simulink model "L4_SIM"  (R2018a)
settings: Solver=ode1  StartTime=0.0  StopTime=60  FixedStep=GLB_FIXED_STEP_SIZE_CPV  RelTol=1e-3  EnableMultiTasking=on
undefined symbols (not defined in the file or in its folder): Cf, Chassis, Cr, CYCLE_ACC1_2A__AdaptiveCruiseCtrlMode, CYCLE_ACC1_2A__AdaptiveCruiseCtrlSetSpeed, CYCLE_CCVS1_00__CruiseCtrlSetSpeed, CYCLE_CCVS1_00__WheelBasedVehicleSpeed, CYCLE_EEC1_00__EngSpeed, CYCLE_ETC1_00__TransDrivelineEngaged, CYCLE_ETC2_00__TransActualGearRatio, CYCLE_ETC7_03__TransMode1Indicator, CYCLE_GPS_Latitude, CYCLE_GPS_Longitude, CYCLE_LFE1_00__EngFuelRate, CYCLE_Net_Engine_Percent_Torque, CYCLE_SSI2_03__PitchAngleExRange, CYCLE_TIME, CYCLE_UTM_Origin_X, CYCLE_UTM_Origin_Y, CYCLE_Vehicle_Distance, DiscIntNeverNeededParam, ENUM_J1939_PCC_STATE_T, ENUM_J1939_SWITCH_T, ENUM_STEERING_WHEEL_ANGLE_SENSOR_TYPE_T, GLB_FIXED_STEP_SIZE_CPV, GLB_TRANS_LOSS_TRQ_GEAR_STEP_MPV, GLB_TRANS_LOSS_TRQ_SPD_STEP_MPV, GLB_TRANS_LOSS_TRQ_TABLE_DATA_MPV, GLB_TRANS_LOSS_TRQ_TRQ_STEP_MPV, GLB_VEHICLE_CONFIG_ACCEL_PED_GATEWAY_APV, heading_0, Iz, L4_Controller, lf, lr, position_0, ptc_matlab_lib, STEERCTRL_10ms, SUB_ECU_L4_MABX, SUB_L4_Task_10ms, SUB_L4_Task_10ms_SUB_STEERCTRL, SUB_PLANT_Chassis, Task_10ms, Vx_0
libraries: EmE_MBD_Blockset x81, PTC_MBDS_LIB x71, simulink x38, simulink_extras x1, SUB_L4_Task_10000ms x1, SUB_L4_Task_1000ms x1, SUB_L4_Task_100ms x1, SUB_L4_Task_10ms_SUB_APTC x1, SUB_L4_Task_10ms_SUB_BRKPEDARB x1, SUB_L4_Task_10ms_SUB_FAULT_MANAGER x1, SUB_L4_Task_10ms_SUB_STATE_CONTROL x1, simulink_need_slupdate x1
(part 5 of 6)

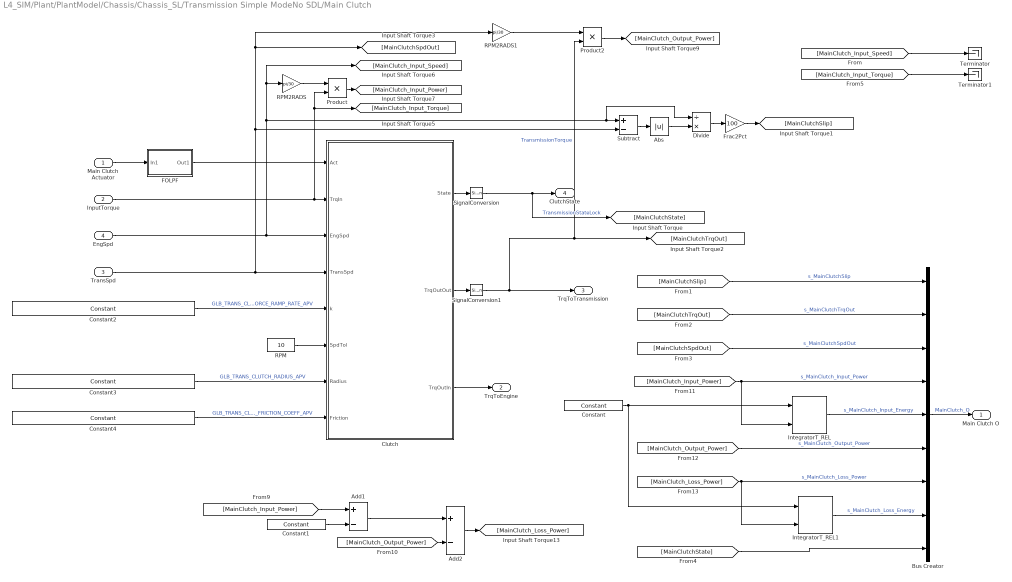
== system L4_SIM/Plant/PlantModel/Chassis/Chassis_SL/Transmission Simple ModeNo SDL/Main Clutch ==
  Main Clutch Actuator : Inport
  InputTorque : Inport  Port=2
  TransSpd : Inport  Port=3
  EngSpd : Inport  Port=4
  Abs : Abs
  Add1 : Sum  Inputs=+-
  Add2 : Sum  Inputs=+-
  Bus Creator : BusCreator  Inputs=9
  Clutch : Stateflow chart  TreatAsAtomicUnit=on
  Constant : PTC_MBDS_LIB/Extras/Sources/Constant  Value2=1  PTC_MBDS_BlockVersion=5.41  PTC_BlockType=PTC_MBDS_Constant
      settings: SourceProductName=PACCAR Technical Center MBDS Library
  Constant1 : PTC_MBDS_LIB/Extras/Sources/Constant  Value2=0  PTC_MBDS_BlockVersion=5.41  PTC_BlockType=PTC_MBDS_Constant
      settings: SourceProductName=PACCAR Technical Center MBDS Library
  Constant2 : PTC_MBDS_LIB/Extras/Sources/Constant  Value2=GLB_TRANS_CLUTCH_FORCE_RAMP_RATE_APV  PTC_MBDS_BlockVersion=5.41  PTC_BlockType=PTC_MBDS_Constant
      settings: SourceProductName=PACCAR Technical Center MBDS Library
      settings: AttributesFormatString=|
      | Value: 5000
      | Unit: 'N/s'
  Constant3 : PTC_MBDS_LIB/Extras/Sources/Constant  Value2=GLB_TRANS_CLUTCH_RADIUS_APV  PTC_MBDS_BlockVersion=5.41  PTC_BlockType=PTC_MBDS_Constant
      settings: SourceProductName=PACCAR Technical Center MBDS Library
      settings: AttributesFormatString=|
      | Value: 0.215
      | Unit: 'm'
  Constant4 : PTC_MBDS_LIB/Extras/Sources/Constant  Value2=GLB_TRANS_CLUTCH_FRICTION_COEFF_APV  PTC_MBDS_BlockVersion=5.41  PTC_BlockType=PTC_MBDS_Constant
      settings: SourceProductName=PACCAR Technical Center MBDS Library
      settings: AttributesFormatString=|
      | Value: 0.3
      | Unit: '1'
  Divide : Product  Inputs=/*
  FOLPF : Subsystem
  Frac2Pct : Gain  Gain=100
  IntegratorT_REL : PTC_MBDS_LIB/MBDS Standard Library/Extended Operations/Integrators/IntegratorT_REL  MXMN_Enabled=off  MX=Inf  MN=-Inf  dT_Enabled=off  dT=GLB_FIXED_STEP_SIZE_CPV  E_Enabled=off  R_Enabled=off  IV_Enabled=off  IV=0  B_min_Enabled=off  B_max_Enabled=off  PTC_MBDS_BlockVersion=5.41  PTC_BlockType=PTC_MBDS_IntegratorT_REL
      settings: SourceProductName=PACCAR Technical Center MBDS Library
      settings: AttributesFormatString=|
      | IV = %<IV>
      | MN = %<MN>
      | MX = %<MX>
      | dT = %<dT>
  IntegratorT_REL1 : PTC_MBDS_LIB/MBDS Standard Library/Extended Operations/Integrators/IntegratorT_REL  MXMN_Enabled=off  MX=Inf  MN=-Inf  dT_Enabled=off  dT=GLB_FIXED_STEP_SIZE_CPV  E_Enabled=off  R_Enabled=off  IV_Enabled=off  IV=0  B_min_Enabled=off  B_max_Enabled=off  PTC_MBDS_BlockVersion=5.41  PTC_BlockType=PTC_MBDS_IntegratorT_REL
      settings: SourceProductName=PACCAR Technical Center MBDS Library
      settings: AttributesFormatString=|
      | IV = %<IV>
      | MN = %<MN>
      | MX = %<MX>
      | dT = %<dT>
  Product : Product  RndMeth=Zero
  Product2 : Product  RndMeth=Zero
  RPM : Constant  Value=10
  RPM2RADS : Gain  Gain=pi/30
  RPM2RADS1 : Gain  Gain=pi/30
  SignalConversion : SignalConversion  ConversionOutput=Contiguous copy  OverrideOpt=off
  SignalConversion1 : SignalConversion  ConversionOutput=Contiguous copy  OverrideOpt=off
  Subtract : Sum  Inputs=+-
  Terminator : Terminator
      settings: InitFcn=|
      | try
      |    MBDS_BlockCallback('Update', gcb);
      | end
  Terminator1 : Terminator
      settings: InitFcn=|
      | try
      |    MBDS_BlockCallback('Update', gcb);
      | end
  Main Clutch O : Outport
  TrqToEngine : Outport  Port=2
  TrqToTransmission : Outport  Port=3
  ClutchState : Outport  Port=4
  wires:
  Constant2/1 -> Clutch/5(k)  "GLB_TRANS_CLUTCH_FORCE_RAMP_RATE_APV"
  SignalConversion1/1 -> TrqToTransmission/1, [MainClutchTrqOut], Product2/2  "TransmissionTorque"
  SignalConversion/1 -> [MainClutchState], ClutchState/1  "TransmissionStateLock"
  [MainClutch_Input_Torque] -> Terminator1/1
  [MainClutch_Input_Speed] -> Terminator/1
  [MainClutchState] -> Bus Creator/9
  Constant1/1 -> Add1/2
  Constant/1 -> IntegratorT_REL/1, IntegratorT_REL1/1
  Constant3/1 -> Clutch/7(Radius)  "GLB_TRANS_CLUTCH_RADIUS_APV"
  Constant4/1 -> Clutch/8(Friction)  "GLB_TRANS_CLUTCH_FRICTION_COEFF_APV"
  TransSpd/1 -> [MainClutchSpdOut], RPM2RADS1/1, Subtract/2, Clutch/4(TransSpd)
  Subtract/1 -> Abs/1
  Abs/1 -> Divide/2
  Divide/1 -> Frac2Pct/1
  RPM2RADS1/1 -> Product2/1
  RPM2RADS/1 -> Product/1
  Clutch/1(State) -> SignalConversion/1
  FOLPF/1(Out1) -> Clutch/1(Act)
  RPM/1 -> Clutch/6(SpdTol)
  EngSpd/1 -> RPM2RADS/1, [MainClutch_Input_Speed], Subtract/1, Divide/1, Clutch/3(EngSpd)
  InputTorque/1 -> [MainClutch_Input_Torque], Product/2, Clutch/2(TrqIn)
  Clutch/2(TrqOutOut) -> SignalConversion1/1
  Clutch/3(TrqOutIn) -> TrqToEngine/1
  Frac2Pct/1 -> [MainClutchSlip]
  [MainClutchSpdOut] -> Bus Creator/3  "s_MainClutchSpdOut"
  [MainClutchTrqOut] -> Bus Creator/2  "s_MainClutchTrqOut"
  [MainClutchSlip] -> Bus Creator/1  "s_MainClutchSlip"
  Bus Creator/1 -> Main Clutch O/1  "MainClutch_O"
  Main Clutch Actuator/1 -> FOLPF/1(In1)
  Product/1 -> [MainClutch_Input_Power]
  Product2/1 -> [MainClutch_Output_Power]
  [MainClutch_Input_Power] -> Add1/1
  [MainClutch_Output_Power] -> Add2/2
  Add1/1 -> Add2/1
  Add2/1 -> [MainClutch_Loss_Power]
  [MainClutch_Input_Power] -> Bus Creator/4, IntegratorT_REL/2  "s_MainClutch_Input_Power"
  [MainClutch_Output_Power] -> Bus Creator/6  "s_MainClutch_Output_Power"
  [MainClutch_Loss_Power] -> Bus Creator/7, IntegratorT_REL1/2  "s_MainClutch_Loss_Power"
  IntegratorT_REL1/1 -> Bus Creator/8  "s_MainClutch_Loss_Energy"
  IntegratorT_REL/1 -> Bus Creator/5  "s_MainClutch_Input_Energy"

== system L4_SIM/Controllers/Operator/Subsystem/SpdControlBrake/SpdControlBrake/PID/AntiWindup ==
  note: NOTE: THE ANTI-WINDUP FOR BRAKE IS THE SAME AS FOR TRACTION EXCEPT
      | FOR THE SAT_STATE LOGIC
  I_update : Inport
  Sat_state : Inport  Port=2
  Constant : Constant  Value=0
  Constant1 : Constant  Value=-1
  Constant2 : Constant
  Constant3 : Constant
  Constant4 : Constant  Value=-1
  Constant5 : Constant  Value=2
  Logical Operator : Logic  Operator=OR  AllPortsSameDT=off  OutDataTypeStr=boolean
  Logical Operator1 : Logic  AllPortsSameDT=off  OutDataTypeStr=boolean
  Logical Operator2 : Logic  AllPortsSameDT=off  OutDataTypeStr=boolean
  Logical Operator3 : Logic  AllPortsSameDT=off  OutDataTypeStr=boolean
  Relational Operator1 : RelationalOperator  Operator=~=  OutDataTypeStr=boolean  RndMeth=Nearest
  Relational Operator2 : RelationalOperator  Operator=~=  OutDataTypeStr=boolean  RndMeth=Nearest
  Relational Operator3 : RelationalOperator  Operator===  OutDataTypeStr=boolean  RndMeth=Nearest
  Relational Operator4 : RelationalOperator  Operator===  OutDataTypeStr=boolean  RndMeth=Nearest
  Relational Operator5 : RelationalOperator  Operator=~=  OutDataTypeStr=boolean  RndMeth=Nearest
  Sign1 : Signum
  Switch1 : Switch  Criteria=u2 ~= 0
  I_update_clp : Outport
  wires:
  Logical Operator1/1 -> Logical Operator/1
  Logical Operator/1 -> Logical Operator3/2
  Relational Operator5/1 -> Logical Operator3/1
  [Sat_state] -> Relational Operator5/1
  Constant5/1 -> Relational Operator5/2
  Logical Operator3/1 -> Switch1/2
  Constant/1 -> Switch1/3
  Logical Operator2/1 -> Logical Operator/2
  Relational Operator1/1 -> Logical Operator2/1
  Relational Operator3/1 -> Logical Operator2/2
  Relational Operator4/1 -> Logical Operator1/1
  Relational Operator2/1 -> Logical Operator1/2
  Constant4/1 -> Relational Operator4/1
  Constant3/1 -> Relational Operator3/1
  Sign1/1 -> Relational Operator3/2, Relational Operator4/2
  Constant2/1 -> Relational Operator2/2
  Sat_state/1 -> [Sat_state], Relational Operator2/1, Relational Operator1/1
  Constant1/1 -> Relational Operator1/2
  I_update/1 -> Switch1/1, Sign1/1
  Switch1/1 -> I_update_clp/1

== system L4_SIM/Controllers/Operator/Subsystem/SpdControlTraction/SpdControlTraction/PID/AntiWindup ==
  I_update : Inport
  Sat_state : Inport  Port=2
  Constant : Constant  Value=0
  Constant1 : Constant
  Constant2 : Constant  Value=-1
  Constant3 : Constant
  Constant4 : Constant  Value=-1
  Constant5 : Constant  Value=2
  Logical Operator : Logic  Operator=OR  AllPortsSameDT=off  OutDataTypeStr=boolean
  Logical Operator1 : Logic  AllPortsSameDT=off  OutDataTypeStr=boolean
  Logical Operator2 : Logic  AllPortsSameDT=off  OutDataTypeStr=boolean
  Logical Operator3 : Logic  AllPortsSameDT=off  OutDataTypeStr=boolean
  Relational Operator1 : RelationalOperator  Operator=~=  OutDataTypeStr=boolean  RndMeth=Nearest
  Relational Operator2 : RelationalOperator  Operator=~=  OutDataTypeStr=boolean  RndMeth=Nearest
  Relational Operator3 : RelationalOperator  Operator===  OutDataTypeStr=boolean  RndMeth=Nearest
  Relational Operator4 : RelationalOperator  Operator===  OutDataTypeStr=boolean  RndMeth=Nearest
  Relational Operator5 : RelationalOperator  Operator=~=  OutDataTypeStr=boolean  RndMeth=Nearest
  Sign1 : Signum
  Switch1 : Switch  Criteria=u2 ~= 0
  I_update_clp : Outport
  wires:
  Relational Operator5/1 -> Logical Operator3/1
  [Sat_state] -> Relational Operator5/1
  Constant5/1 -> Relational Operator5/2
  Logical Operator/1 -> Logical Operator3/2
  Logical Operator3/1 -> Switch1/2
  Constant/1 -> Switch1/3
  Logical Operator2/1 -> Logical Operator/2
  Logical Operator1/1 -> Logical Operator/1
  Relational Operator1/1 -> Logical Operator2/1
  Relational Operator3/1 -> Logical Operator2/2
  Relational Operator4/1 -> Logical Operator1/1
  Relational Operator2/1 -> Logical Operator1/2
  Constant4/1 -> Relational Operator4/1
  Constant3/1 -> Relational Operator3/1
  Sign1/1 -> Relational Operator3/2, Relational Operator4/2
  Constant2/1 -> Relational Operator2/2
  Sat_state/1 -> [Sat_state], Relational Operator2/1, Relational Operator1/1
  Constant1/1 -> Relational Operator1/2
  I_update/1 -> Switch1/1, Sign1/1
  Switch1/1 -> I_update_clp/1

== system L4_SIM/Controllers/Virtual_Controllers/L4_MABX/L4_Controller/Task_10ms/STEERCTRL_10ms/LPF ==
  In1 : Inport
  Constant : Constant  Value=0.1
  Constant1 : Constant  Value=ptc_matlab_lib.get_system_sample_time()
  LowpassT_RE : PTC_MBDS_LIB/MBDS Standard Library/Extended Operations/Filters/LowpassT_RE  dT_Enabled=on  dT=ptc_matlab_lib.get_system_sample_time()  E_Enabled=off  R_Enabled=off  IV_Enabled=off  IV=0  PTC_MBDS_BlockVersion=5.41  PTC_BlockType=PTC_MBDS_LowpassT_RE
      settings: AttributesFormatString=IV = %<IV>  SourceProductName=PACCAR Technical Center MBDS Library
  Out1 : Outport
  wires:
  In1/1 -> LowpassT_RE/3
  LowpassT_RE/1 -> Out1/1
  Constant/1 -> LowpassT_RE/1
  Constant1/1 -> LowpassT_RE/2

== system L4_SIM/Controllers/Virtual_Controllers/L4_MABX/L4_Controller/Task_10ms/STEERCTRL_10ms/LPF1 ==
  In1 : Inport
  Constant : Constant  Value=2.0
  Constant1 : Constant  Value=0.01
  Data Type Conversion : DataTypeConversion  OutDataTypeStr=boolean  SaturateOnIntegerOverflow=on
  LowpassT_RE : PTC_MBDS_LIB/MBDS Standard Library/Extended Operations/Filters/LowpassT_RE  dT_Enabled=on  dT=ptc_matlab_lib.get_system_sample_time()  E_Enabled=off  R_Enabled=on  IV_Enabled=off  IV=0  PTC_MBDS_BlockVersion=5.41  PTC_BlockType=PTC_MBDS_LowpassT_RE
      settings: AttributesFormatString=IV = %<IV>  SourceProductName=PACCAR Technical Center MBDS Library
  Step : Step  Time=ptc_matlab_lib.get_system_sample_time()  Before=1  After=0
  Out1 : Outport
  wires:
  Constant1/1 -> LowpassT_RE/2
  Data Type Conversion/1 -> LowpassT_RE/4
  Step/1 -> Data Type Conversion/1
  Constant/1 -> LowpassT_RE/1
  LowpassT_RE/1 -> Out1/1
  In1/1 -> LowpassT_RE/3

== system L4_SIM/Controllers/Virtual_Controllers/L4_MABX/L4_Controller/Task_10ms/STEERCTRL_10ms/PID ==
  err : Inport
  kp : Inport  Port=2
  Constant19 : Constant  Value=240
  Constant20 : Constant  Value=-240
  Constant21 : Constant  Value=.01
  Constant8 : Constant  Value=boolean(0)
  Constant9 : Constant  Value=0
  PID : Subsystem
  SteeringControlDGain : Constant  Value=.01
  SteeringControlIntGain : Constant  Value=20
  Out1 : Outport
  Out2 : Outport  Port=2
  Out3 : Outport  Port=3
  Out4 : Outport  Port=4
  wires:
  SteeringControlDGain/1 -> PID/4(Td)
  SteeringControlIntGain/1 -> PID/3(Ti)
  PID/1(Y) -> Out1/1
  PID/2(P) -> Out2/1
  PID/4(D) -> Out4/1
  PID/3(I) -> Out3/1
  Constant8/1 -> PID/5(Reset_f)
  Constant21/1 -> PID/6(Ts)
  Constant19/1 -> PID/7(UpperLim)
  Constant20/1 -> PID/8(LowerLim)
  Constant9/1 -> PID/9(InitOutput)
  kp/1 -> PID/2(Kp)
  err/1 -> PID/1(Err)

== system L4_SIM/Controllers/Virtual_Controllers/L4_MABX/L4_Controller/Task_10ms/STEERCTRL_10ms/SteerController ==
  note: Generate a 0.1-1.0 scale factor based on inverse of imput speed
  MeasuredHeading : Inport
  RefHeading : Inport  Port=2
  TrackingSignal : Inport  Port=3
  FrontAxelSpeed : Inport  Port=4
  0.1-0.01 : Math  Operator=reciprocal  SaturateOnIntegerOverflow=on
  10kph-100kph : Saturate  UpperLimit=100  LowerLimit=10
  Command : Scope  NumInputPorts=2
  Error Calc : MATLAB Function  TreatAsAtomicUnit=on
  Gain1 : Gain  Gain=-1
  Gain2 : Gain  Gain=10
  Lateral Controller : simulink/Continuous/PID Controller  Controller=PID  TimeDomain=Discrete-time  SampleTime=-1  IntegratorMethod=Forward Euler  FilterMethod=Forward Euler  Form=Parallel  UseFilter=on  ControllerParametersSource=internal  P=4  I=0.25  D=0.1  N=100  InitialConditionSource=internal  InitialConditionForIntegrator=0  InitialConditionForFilter=0  ExternalReset=none  LimitOutput=on  UpperSaturationLimit=0.5  LowerSaturationLimit=-0.5  LinearizeAsGain=on  AntiWindupMode=back-calculation  Kb=1  TrackingMode=on  Kt=1  PParamMin=[]  PParamMax=[]  IParamMin=[]  IParamMax=[]  DParamMin=[]  DParamMax=[]  NParamMin=[]  NParamMax=[]  KbParamMin=[]  KbParamMax=[]  KtParamMin=[]  KtParamMax=[]  POutMin=[]  POutMax=[]  IOutMin=[]  IOutMax=[]  DOutMin=[]  DOutMax=[]  NOutMin=[]  NOutMax=[]  KbOutMin=[]  KbOutMax=[]  KtOutMin=[]  KtOutMax=[]  IntegratorOutMin=[]  IntegratorOutMax=[]  FilterOutMin=[]  FilterOutMax=[]  SumOutMin=[]  SumOutMax=[]  SumI1OutMin=[]  SumI1OutMax=[]  SumI2OutMin=[]  SumI2OutMax=[]  SumI3OutMin=[]  SumI3OutMax=[]  SumDOutMin=[]  SumDOutMax=[]  SaturationOutMin=[]  SaturationOutMax=[]  IntegratorContinuousStateAttributes=''  IntegratorStateMustResolveToSignalObject=off  IntegratorRTWStateStorageClass=Auto  FilterContinuousStateAttributes=''  FilterStateMustResolveToSignalObject=off  FilterRTWStateStorageClass=Auto  DifferentiatorICPrevScaledInput=0  DifferentiatorOutMin=[]  DifferentiatorOutMax=[]  FilterDiffOutCoefMin=[]  FilterDiffOutCoefMax=[]  SumDenOutMin=[]  SumDenOutMax=[]  SumNumOutMin=[]  SumNumOutMax=[]  ReciprocalOutMin=[]  ReciprocalOutMax=[]  DivideOutMin=[]  DivideOutMax=[]  TunerSelectOption=Transfer Function Based (PID Tuner App)
  Max Axel Angle : Gain  Gain=5
  Rate Limiter : RateLimiter  RisingSlewLimit=0.1  FallingSlewLimit=-0.1  SampleTimeMode=inherited
  Saturation Dynamic : simulink/Discontinuities/Saturation Dynamic  OutMin=[]  OutMax=[]  OutDataTypeStr=Inherit: Same as second input  OutDataType=fixdt(1, 16)  OutScaling=2^-10  DoSatur=off
  SteerCommand : Outport
  wires:
  MeasuredHeading/1 -> Error Calc/1(current)
  RefHeading/1 -> Error Calc/2(target)
  Error Calc/1(error) -> Command/1, Lateral Controller/1  "heading error"
  TrackingSignal/1 -> Lateral Controller/2
  Gain2/1 -> Max Axel Angle/1
  0.1-0.01/1 -> Gain2/1
  10kph-100kph/1 -> 0.1-0.01/1
  FrontAxelSpeed/1 -> 10kph-100kph/1
  Lateral Controller/1 -> Command/2, Saturation Dynamic/2  "Steer Command"
  Max Axel Angle/1 -> Gain1/1, Saturation Dynamic/1
  Gain1/1 -> Saturation Dynamic/3
  Rate Limiter/1 -> SteerCommand/1
  Saturation Dynamic/1 -> Rate Limiter/1

== system L4_SIM/Controllers/Virtual_Controllers/L4_MABX/L4_Controller/Task_10ms/STEERCTRL_10ms/ValidateError ==
  error : Inport
  Abs : Abs
  Add : Sum  Inputs=-+
  Data Type Conversion : DataTypeConversion  OutDataTypeStr=boolean
  Detect Change : simulink/Logic and Bit Operations/Detect Change  vinit=0  InputProcessing=Inherited  OutDataTypeStr=boolean
  JumpNearEdge : Logic  AllPortsSameDT=off  OutDataTypeStr=boolean
  LPF_first_order : EmE_MBD_Blockset/Discrete/LPF_first_order
      settings: SourceProductName=PACCAR EmE MBD Blockset
  Product : Product
  Sign : Signum
  Switch : Switch  Criteria=u2 ~= 0
  Switch1 : Switch  Criteria=u2 ~= 0
  closeToEdge : RelationalOperator  Operator=>  OutDataTypeStr=boolean  RndMeth=Nearest
  closeToLaneEdgeThreshold : Constant  Value=4.0
  corrected Error : Sum
  correction : Constant  Value=0.5
  correctionApplied : EmE_MBD_Blockset/Discrete/LPF_first_order
      settings: SourceProductName=PACCAR EmE MBD Blockset
  correctionApplied1 : EmE_MBD_Blockset/Discrete/LPF_first_order
      settings: SourceProductName=PACCAR EmE MBD Blockset
  highRateOfChange : RelationalOperator  Operator=>  OutDataTypeStr=boolean  RndMeth=Nearest
  rateOfChangeThreshold : Constant  Value=5.75
  timeConstant : Constant  Value=1.0
  timeConstant1 : Constant  Value=.01
  timeConstant2 : Constant  Value=3
  timeConstant3 : Constant  Value=.01
  timeConstant4 : Constant  Value=.5
  timeConstant5 : Constant  Value=.01
  zero : Constant  Value=boolean(0)
  zero1 : Constant  Value=0
  zero2 : Constant  Value=0
  zero3 : Constant  Value=boolean(0)
  Out1 : Outport
  wires:
  Abs/1 -> Add/2, closeToEdge/1
  closeToLaneEdgeThreshold/1 -> closeToEdge/2
  zero/1 -> LPF_first_order/1
  timeConstant/1 -> LPF_first_order/4
  timeConstant1/1 -> LPF_first_order/5
  LPF_first_order/1 -> Add/1
  Add/1 -> highRateOfChange/1
  rateOfChangeThreshold/1 -> highRateOfChange/2
  highRateOfChange/1 -> JumpNearEdge/1
  closeToEdge/1 -> JumpNearEdge/2
  JumpNearEdge/1 -> Detect Change/1, Switch1/2, Switch/2
  zero1/1 -> Switch/3
  correction/1 -> Switch/1
  zero2/1 -> correctionApplied/3
  Detect Change/1 -> Data Type Conversion/1
  Switch/1 -> correctionApplied/2
  timeConstant2/1 -> correctionApplied/4
  timeConstant3/1 -> correctionApplied/5
  correctionApplied/1 -> Product/1
  Sign/1 -> Product/2
  Product/1 -> corrected Error/1
  corrected Error/1 -> Out1/1
  Data Type Conversion/1 -> correctionApplied/1
  zero3/1 -> correctionApplied1/1
  error/1 -> Sign/1, correctionApplied1/3, correctionApplied1/2, Switch1/3, LPF_first_order/3, LPF_first_order/2, Abs/1
  timeConstant4/1 -> correctionApplied1/4
  timeConstant5/1 -> correctionApplied1/5
  correctionApplied1/1 -> Switch1/1
  Switch1/1 -> corrected Error/2

== system L4_SIM/Controllers/Virtual_Controllers/L4_MABX/L4_Controller/Task_10ms/STEERCTRL_10ms/slew ==
  numLanePoints : Inport
  rawError : Inport  Port=2
  Chart : Stateflow chart  TreatAsAtomicUnit=on
  Constant : Constant  Value=uint8(3)
  Constant1 : Constant  Value=0
  Constant2 : Constant  Value=.01
  Constant3 : Constant  Value=2
  Constant4 : Constant  Value=-2
  Data Type Conversion : DataTypeConversion  OutDataTypeStr=boolean
  Relational Operator : RelationalOperator  OutDataTypeStr=boolean  RndMeth=Nearest
  Slew_at_event : EmE_MBD_Blockset/Math Operators/Slew_at_event
      settings: SourceProductName=PACCAR EmE MBD Blockset
  Switch : Switch  Criteria=u2 ~= 0
  Switch1 : Switch  Criteria=u2 ~= 0
  Terminator : Terminator
  enable : Constant
  enableSlew : Constant
  slewedError : Outport
  wires:
  Slew_at_event/1 -> Terminator/1
  enable/1 -> Slew_at_event/Enable
  Slew_at_event/2 -> Switch1/1
  numLanePoints/1 -> Relational Operator/1, Chart/1(numLanePoints)
  Chart/1(stateChange) -> Data Type Conversion/1
  Constant/1 -> Relational Operator/2
  Constant1/1 -> Switch/3
  rawError/1 -> Switch/1
  Relational Operator/1 -> Switch/2
  Switch/1 -> Switch1/3, Slew_at_event/2, Slew_at_event/3
  Constant2/1 -> Slew_at_event/6
  Constant3/1 -> Slew_at_event/4
  Constant4/1 -> Slew_at_event/5
  Data Type Conversion/1 -> Slew_at_event/1
  Switch1/1 -> slewedError/1
  enableSlew/1 -> Switch1/2

== system L4_SIM/Controllers/Virtual_Controllers/L4_MABX/L4_Controller/Task_10ms/STEERCTRL_10ms/stanley ==
  note: At 400 this starts to go unstable on HS track at 300 misses one curve on Dura
  note: Stanley Steering Control
  crossTrackError : Inport
  vehSpeed_kph : Inport  Port=2
  desPathHeading_rad : Inport  Port=3
  steerTireAngle_rad : Inport  Port=4
  1-D Lookup Table : Lookup_n-D  NumberOfTableDimensions=1  BreakpointsForDimension1=[0 5 10 15 25 35 45 55 65]  Table=[.1 .5 .9 1 1 1 .9 .8 .7]  InternalRulePriority=Speed  RndMeth=Simplest  InputSameDT=on
  Add1 : Sum
  Add2 : Sum  Inputs=+-
  AdjustedStanleyGain : Product
  Product : Product
  Saturation : Saturate  UpperLimit=255  LowerLimit=7.5
  Trigonometric Function : Trigonometry  Operator=atan2
  desHeadingWeight : Gain  Gain=0
  kph2mps_ : Gain  Gain=1/3.6  OutDataTypeStr=double
  stanleySteeringControlGain : Constant  Value=double(350)
  desSteeringAngle : Outport
  wires:
  Add1/1 -> desSteeringAngle/1
  AdjustedStanleyGain/1 -> Product/1
  Product/1 -> Trigonometric Function/1
  kph2mps_/1 -> Trigonometric Function/2
  vehSpeed_kph/1 -> 1-D Lookup Table/1, Saturation/1
  Trigonometric Function/1 -> Add1/1
  Add2/1 -> desHeadingWeight/1
  crossTrackError/1 -> Product/2
  steerTireAngle_rad/1 -> Add2/1
  desPathHeading_rad/1 -> Add2/2
  desHeadingWeight/1 -> Add1/2
  Saturation/1 -> kph2mps_/1
  stanleySteeringControlGain/1 -> AdjustedStanleyGain/2
  1-D Lookup Table/1 -> AdjustedStanleyGain/1

== system L4_SIM/Controllers/Virtual_Controllers/L4_MABX/L4_Controller/Task_10ms/Vehicle_speed_target/Determine_linear_vehicle_speed_profile ==
  Vehicle_speed : Inport
  Vehicle_speed_target : Inport  Port=2
  Distance_m : Inport  Port=3
  dT : Inport  Port=4
  Detect Change1 : simulink/Logic and Bit Operations/Detect Change  vinit=0  InputProcessing=Inherited  OutDataTypeStr=boolean
      settings: AttributesFormatString=IC: %<vinit>
  Determine_slew_time_values : Subsystem
  Logical Operator : EmE_MBD_Blockset/Logic and Bit Operations/Logical Operator  Operator=OR  Inputs=1
      settings: SourceProductName=PACCAR EmE MBD Blockset
  Mux : Mux  Inputs=2
  Slew_init_reset : EmE_MBD_Blockset/Math Operators/Slew_init_reset
      settings: SourceProductName=PACCAR EmE MBD Blockset
  Vehicle_speed_profile_linear : Outport  OutputWhenDisabled=reset
  wires:
  dT/1 -> Slew_init_reset/6, Determine_slew_time_values/5(dT)
  Slew_init_reset/1 -> Vehicle_speed_profile_linear/1  "Vehicle_speed_profile_linear"
  Detect Change1/1 -> Logical Operator/1
  Mux/1 -> Detect Change1/1
  Logical Operator/1 -> Determine_slew_time_values/1(F_Reset), Slew_init_reset/1
  Vehicle_speed_target/1 -> Determine_slew_time_values/3(Vehicle_speed_target), Slew_init_reset/3, Mux/2
  Distance_m/1 -> Determine_slew_time_values/4(Distance_m), Mux/1
  Vehicle_speed/1 -> Determine_slew_time_values/2(Vehicle_speed), Slew_init_reset/2
  Determine_slew_time_values/1(Inc) -> Slew_init_reset/4
  Determine_slew_time_values/2(Dec) -> Slew_init_reset/5

== system L4_SIM/Controllers/Virtual_Controllers/L4_MABX/L4_Controller/Task_10ms/Vehicle_speed_target/Determine_sigmoid_vehicle_speed_profile ==
  F_Enable : Inport
  Distance_m : Inport  Port=2
  Vehicle_speed : Inport  Port=3
  Vehicle_speed_target : Inport  Port=4
  Vehicle_acceleration : Inport  Port=5
  Vehicle_acceleration_target : Inport  Port=6
  Jerk_magnitude_initial : Inport  Port=7
  Jerk_magnitude_final : Inport  Port=8
  Determine_inhibit_sigmoid_vehicle_speed_profile : Subsystem
  Gain1 : Gain  Gain=1/3.6
  Gain2 : Gain  Gain=1/3.6
  Gain3 : Gain  Gain=3.6
  MIN_VSPD_SIGMOID_FINAL_KPH_APV : EmE_MBD_Blockset/Sources/APV  conval=0
      settings: SourceProductName=PACCAR EmE MBD Blockset
  MIN_VSPD_SIGMOID_INITIAL_KPH_APV : EmE_MBD_Blockset/Sources/APV  conval=5
      settings: SourceProductName=PACCAR EmE MBD Blockset
  MinMax1 : MinMax  Function=max  Inputs=2  InputSameDT=on
  MinMax6 : MinMax  Function=max  Inputs=2  InputSameDT=on
  Saturation1 : Saturate  UpperLimit=10  LowerLimit=0.001
      settings: AttributesFormatString=|
      | Min: %<LowerLimit>
      | Max: %<UpperLimit>
  Saturation2 : Saturate  UpperLimit=10  LowerLimit=0.001
      settings: AttributesFormatString=|
      | Min: %<LowerLimit>
      | Max: %<UpperLimit>
  Saturation4 : Saturate  UpperLimit=255  LowerLimit=0
      settings: AttributesFormatString=|
      | Min: %<LowerLimit>
      | Max: %<UpperLimit>
  Saturation5 : Saturate  UpperLimit=255  LowerLimit=0
      settings: AttributesFormatString=|
      | Min: %<LowerLimit>
      | Max: %<UpperLimit>
  Saturation6 : Saturate  UpperLimit=15.562  LowerLimit=-15.562
      settings: AttributesFormatString=|
      | Min: %<LowerLimit>
      | Max: %<UpperLimit>
  Saturation7 : Saturate  UpperLimit=15.562  LowerLimit=-15.562
      settings: AttributesFormatString=|
      | Min: %<LowerLimit>
      | Max: %<UpperLimit>
  Select_vehicle_speed_target_value : Subsystem
  Terminator : Terminator
  TwentyPointVectorCalculation : Stateflow chart  TreatAsAtomicUnit=on
  VehicleSpeedSetpointDynamicCalculation : Stateflow chart  TreatAsAtomicUnit=on
  F_Inhibit_sigmoid_vector_shaping : Outport  LibraryBlock=EmE_MBD_Blockset/Sinks/Out  OutputWhenDisabled=reset
  Vehicle_speed_profile_sigmoid : Outport  Port=2
  wires:
  Saturation2/1 -> VehicleSpeedSetpointDynamicCalculation/8(JerkMagnitudeFinal)
  Saturation1/1 -> VehicleSpeedSetpointDynamicCalculation/7(JerkMagnitudeInitial)
  Saturation7/1 -> VehicleSpeedSetpointDynamicCalculation/6(AccelerationFinal)
  Saturation6/1 -> VehicleSpeedSetpointDynamicCalculation/5(AccelerationInitial)
  Vehicle_speed_target/1 -> Saturation4/1
  Saturation5/1 -> Determine_inhibit_sigmoid_vehicle_speed_profile/3(Vehicle_speed), Select_vehicle_speed_target_value/4(Vehicle_speed), MinMax6/1
  Saturation4/1 -> Determine_inhibit_sigmoid_vehicle_speed_profile/4(Vehicle_speed_target), Select_vehicle_speed_target_value/5(Vehicle_speed_target), MinMax1/1  "VSPD_TARGET_KPH_APV"
  Determine_inhibit_sigmoid_vehicle_speed_profile/2(Vehicle_speed_initial) -> Select_vehicle_speed_target_value/1(Vehicle_speed_initial)
  MinMax6/1 -> Gain1/1
  MinMax1/1 -> Gain2/1
  MIN_VSPD_SIGMOID_FINAL_KPH_APV/1 -> Select_vehicle_speed_target_value/9(MIN_VSPD_SIGMOID_FINAL_KPH_APV), MinMax1/2
  MIN_VSPD_SIGMOID_INITIAL_KPH_APV/1 -> Select_vehicle_speed_target_value/8(MIN_VSPD_SIGMOID_INITIAL_KPH_APV), MinMax6/2
  Jerk_magnitude_final/1 -> Saturation2/1
  Jerk_magnitude_initial/1 -> Saturation1/1
  VehicleSpeedSetpointDynamicCalculation/3(VelocityVectorRaw) -> TwentyPointVectorCalculation/5(VelocityVectorRaw)
  TwentyPointVectorCalculation/2(PositionVector) -> Select_vehicle_speed_target_value/6(Position_vector_m), Determine_inhibit_sigmoid_vehicle_speed_profile/5(Position_vector_m)  "Position_vector_m"
  VehicleSpeedSetpointDynamicCalculation/1(TimeVectorRaw) -> TwentyPointVectorCalculation/3(TimeVectorRaw)
  TwentyPointVectorCalculation/5(JerkVector) -> Determine_inhibit_sigmoid_vehicle_speed_profile/8(Jerk_vector_ms3)  "Jerk_vector_ms"
  VehicleSpeedSetpointDynamicCalculation/2(PositionVectorRaw) -> TwentyPointVectorCalculation/4(PositionVectorRaw)
  TwentyPointVectorCalculation/4(AccelerationVector) -> Determine_inhibit_sigmoid_vehicle_speed_profile/7(Acceleration_vector_ms2)  "Acceleration_vector_ms"
  VehicleSpeedSetpointDynamicCalculation/4(AccelerationVectorRaw) -> TwentyPointVectorCalculation/6(AccelerationVectorRaw)
  TwentyPointVectorCalculation/3(VelocityVector) -> Gain3/1
  TwentyPointVectorCalculation/1(TimeVector) -> Terminator/1  "Time_vector_secs"
  VehicleSpeedSetpointDynamicCalculation/5(JerkVectorRaw) -> TwentyPointVectorCalculation/7(JerkVectorRaw)
  Select_vehicle_speed_target_value/1(Vehicle_speed_profile_sigmoid) -> Vehicle_speed_profile_sigmoid/1
  Vehicle_speed/1 -> Saturation5/1
  Determine_inhibit_sigmoid_vehicle_speed_profile/1(F_Inhibit_sigmoid_vector_shaping) -> F_Inhibit_sigmoid_vector_shaping/1
  Vehicle_acceleration_target/1 -> Saturation7/1
  Gain3/1 -> Select_vehicle_speed_target_value/7(Vehicle_speed_vector_kph), Determine_inhibit_sigmoid_vehicle_speed_profile/6(Vehicle_speed_vector_kph)  "Vehicle_speed_vector_kph"
  Vehicle_acceleration/1 -> Saturation6/1
  Gain1/1 -> VehicleSpeedSetpointDynamicCalculation/3(VelocityInitial)
  Gain2/1 -> VehicleSpeedSetpointDynamicCalculation/4(VelocityFinal)
  Distance_m/1 -> Determine_inhibit_sigmoid_vehicle_speed_profile/2(Distance_m), Select_vehicle_speed_target_value/3(Distance_m), TwentyPointVectorCalculation/2(PositionFinal), VehicleSpeedSetpointDynamicCalculation/2(PositionFinal)
  F_Enable/1 -> Determine_inhibit_sigmoid_vehicle_speed_profile/1(F_Enable), Select_vehicle_speed_target_value/2(F_Enable), TwentyPointVectorCalculation/1(Enable), VehicleSpeedSetpointDynamicCalculation/1(Enable)

== system L4_SIM/Controllers/Virtual_Controllers/L4_MABX/L4_Controller/Task_10ms/Vehicle_speed_target/Forward collision warning speed limit ==
  In : Inport
  Bus Selector1 : BusSelector  OutputSignals=CAN.EBC2_0B.FrontAxleSpeed,CAN.ACC1_2A.ACCDistanceAlertSignal,CAN.ACC1_2A.ForwardCollisionWarning
  Compare To Constant3 : simulink/Logic and Bit Operations/Compare To Constant  relop===  const=1  OutDataTypeStr=boolean
  Compare To Constant8 : simulink/Logic and Bit Operations/Compare To Constant  relop===  const=1  OutDataTypeStr=boolean
  Constant4 : Constant  Value=255
  FCW_ACTIVE_VSPD_TARGET_APV : Constant  Value=0
  FCW_CTRL_SLEW_DEC_APV : Constant  Value=5000
  FCW_CTRL_SLEW_INC_APV : Constant
  If_Then_Else4 : EmE_MBD_Blockset/Signal Routing/If_Then_Else
      settings: SourceProductName=PACCAR EmE MBD Blockset
  Logical Operator1 : Logic  Operator=OR  OutDataTypeStr=boolean
  MinMax : MinMax  Inputs=2  InputSameDT=on
  Rising_edge : EmE_MBD_Blockset/Discontinuities/Rising_edge  initact=off
      settings: AttributesFormatString=Action on IC: %<initact>  SourceProductName=PACCAR EmE MBD Blockset
  Slew_init_reset : EmE_MBD_Blockset/Math Operators/Slew_init_reset
      settings: SourceProductName=PACCAR EmE MBD Blockset
  Unit_Delay : UnitDelay  SampleTime=-1
      settings: AttributesFormatString=IC: %<vinit>
  dT : EmE_MBD_Blockset/Sources/dT
      settings: SourceProductName=PACCAR EmE MBD Blockset
  FCW_vehicle_speed_limit : Outport
  wires:
  In/1 -> Bus Selector1/1
  Compare To Constant3/1 -> Logical Operator1/1
  Bus Selector1/2 -> Compare To Constant3/1  "<ACCDistanceAlertSignal>"
  Compare To Constant8/1 -> Logical Operator1/2
  Bus Selector1/3 -> Compare To Constant8/1  "<ForwardCollisionWarning>"
  Rising_edge/1 -> Slew_init_reset/1
  Unit_Delay/1 -> MinMax/1
  If_Then_Else4/1 -> Slew_init_reset/3
  Logical Operator1/1 -> If_Then_Else4/1, Rising_edge/1
  dT/1 -> Slew_init_reset/6
  Constant4/1 -> If_Then_Else4/3
  Bus Selector1/1 -> MinMax/2  "<FrontAxleSpeed>"
  Slew_init_reset/1 -> FCW_vehicle_speed_limit/1, Unit_Delay/1  "FCW_vehicle_speed_limit"
  FCW_CTRL_SLEW_DEC_APV/1 -> Slew_init_reset/5
  FCW_ACTIVE_VSPD_TARGET_APV/1 -> If_Then_Else4/2
  FCW_CTRL_SLEW_INC_APV/1 -> Slew_init_reset/4
  MinMax/1 -> Slew_init_reset/2

== system L4_SIM/Controllers/Virtual_Controllers/L4_MABX/L4_Controller/Task_10ms/Vehicle_speed_target/Stability control speed limit ==
  In : Inport
  Bus Selector5 : BusSelector  OutputSignals=CAN.EBC2_0B.FrontAxleSpeed,CAN.VDC1_0B.ROPEngCtrlActive,CAN.VDC1_0B.ROPBrakeCtrlActive,CAN.VDC1_0B.YCEngCtrlActive,CAN.VDC1_0B.YCBrakeCtrlActive
  Compare To Constant{9..12} (4 alike) : simulink/Logic and Bit Operations/Compare To Constant  relop===  const=1  OutDataTypeStr=boolean
  Constant4 : Constant  Value=255
  If_Then_Else4 : EmE_MBD_Blockset/Signal Routing/If_Then_Else
      settings: SourceProductName=PACCAR EmE MBD Blockset
  Logical Operator2 : Logic  Operator=OR  Inputs=4  OutDataTypeStr=boolean
  MinMax : MinMax  Inputs=2  InputSameDT=on
  Rising_edge : EmE_MBD_Blockset/Discontinuities/Rising_edge  initact=off
      settings: AttributesFormatString=Action on IC: %<initact>  SourceProductName=PACCAR EmE MBD Blockset
  STABILITY_ACTIVE_VSPD_TARGET_APV : Constant  Value=0
  STABILITY_CTRL_SLEW_DEC_APV : Constant  Value=5
  STABILITY_CTRL_SLEW_INC_APV : Constant  Value=3
  Slew_init_reset : EmE_MBD_Blockset/Math Operators/Slew_init_reset
      settings: SourceProductName=PACCAR EmE MBD Blockset
  Unit_Delay : UnitDelay  SampleTime=-1
      settings: AttributesFormatString=IC: %<vinit>
  dT : EmE_MBD_Blockset/Sources/dT
      settings: SourceProductName=PACCAR EmE MBD Blockset
  Stability_control_vehicle_speed_limit : Outport
  wires:
  Bus Selector5/4 -> Compare To Constant11/1  "<YCEngCtrlActive>"
  Bus Selector5/2 -> Compare To Constant9/1  "<ROPEngCtrlActive>"
  Bus Selector5/5 -> Compare To Constant12/1  "<YCBrakeCtrlActive>"
  Compare To Constant10/1 -> Logical Operator2/2
  Compare To Constant12/1 -> Logical Operator2/4
  Compare To Constant9/1 -> Logical Operator2/1
  Compare To Constant11/1 -> Logical Operator2/3
  dT/1 -> Slew_init_reset/6
  Constant4/1 -> If_Then_Else4/3
  STABILITY_CTRL_SLEW_INC_APV/1 -> Slew_init_reset/4
  STABILITY_CTRL_SLEW_DEC_APV/1 -> Slew_init_reset/5
  STABILITY_ACTIVE_VSPD_TARGET_APV/1 -> If_Then_Else4/2
  If_Then_Else4/1 -> Slew_init_reset/3
  In/1 -> Bus Selector5/1
  Bus Selector5/3 -> Compare To Constant10/1  "<ROPBrakeCtrlActive>"
  Logical Operator2/1 -> If_Then_Else4/1, Rising_edge/1
  Slew_init_reset/1 -> Stability_control_vehicle_speed_limit/1, Unit_Delay/1  "Stability_control_vehicle_speed_limit"
  Rising_edge/1 -> Slew_init_reset/1
  MinMax/1 -> Slew_init_reset/2
  Bus Selector5/1 -> MinMax/2  "<FrontAxleSpeed>"
  Unit_Delay/1 -> MinMax/1

== system L4_SIM/Plant/PlantModel/Chassis/Chassis_SL/Chassis/Vehicle Dynamics/Aero ==
  note: Density
      | of Air
  Rho : Inport
  Cd : Inport  Port=2
  Af : Inport  Port=3
  xDot : Inport  Port=4
  Gain3 : Gain  Gain=0.5
  Product : Product
  Product2 : Product
  Product3 : Product
  Signed square : Subsystem
      mask Display: fprintf('Signed\nsquare')
  AeroDragForce : Outport
  wires:
  Af/1 -> Product3/1
  Product2/1 -> Product3/2
  Cd/1 -> Product2/1
  Product/1 -> Product2/2
  Rho/1 -> Product/1
  Signed square/1(Out1) -> Gain3/1
  Gain3/1 -> Product/2
  Product3/1 -> AeroDragForce/1
  xDot/1 -> Signed square/1(In1)

== system L4_SIM/Plant/PlantModel/Chassis/Chassis_SL/Transmission Simple ModeNo SDL/Gears/FrontBoxGear1 ==
  In1 : Inport
  Abs : Abs
  Constant : PTC_MBDS_LIB/Extras/Sources/Constant  Value2=0.2  PTC_MBDS_BlockVersion=5.41  PTC_BlockType=PTC_MBDS_Constant
      settings: SourceProductName=PACCAR Technical Center MBDS Library
  LowpassT_RE : PTC_MBDS_LIB/MBDS Standard Library/Extended Operations/Filters/LowpassT_RE  dT_Enabled=off  dT=GLB_FIXED_STEP_SIZE_CPV  E_Enabled=off  R_Enabled=off  IV_Enabled=off  IV=0  PTC_MBDS_BlockVersion=5.41  PTC_BlockType=PTC_MBDS_LowpassT_RE
      settings: SourceProductName=PACCAR Technical Center MBDS Library
      settings: AttributesFormatString=|
      | IV = %<IV>
      | dT = %<dT>
  Relational Operator : RelationalOperator  OutDataTypeStr=boolean  RndMeth=Nearest
  Saturation : Saturate  UpperLimit=inf  LowerLimit=.1
  Subtract : Sum  Inputs=-+
  TransMdlMaxRatDelta : Constant  Value=.01
  Out1 : Outport
  Diff_F : Outport  Port=2
  wires:
  Constant/1 -> LowpassT_RE/1
  In1/1 -> Subtract/2, LowpassT_RE/2
  LowpassT_RE/1 -> Saturation/1, Subtract/1
  Saturation/1 -> Out1/1
  Relational Operator/1 -> Diff_F/1
  TransMdlMaxRatDelta/1 -> Relational Operator/2
  Abs/1 -> Relational Operator/1
  Subtract/1 -> Abs/1

== system L4_SIM/Plant/PlantModel/Chassis/Chassis_SL/Transmission Simple ModeNo SDL/Main Clutch/FOLPF ==
  In1 : Inport
  Add1 : Sum  Inputs=+-
  Add2 : Sum
  Constant : Constant  Value=.95
  Constant1 : Constant
  Product : Product
  Product1 : Product
  Unit Delay : UnitDelay  SampleTime=-1
  Out1 : Outport
  wires:
  Add2/1 -> Unit Delay/1, Out1/1
  Constant/1 -> Product1/1, Add1/2
  Unit Delay/1 -> Product1/2
  Product1/1 -> Add2/2
  In1/1 -> Product/1
  Product/1 -> Add2/1
  Add1/1 -> Product/2
  Constant1/1 -> Add1/1

== system L4_SIM/Controllers/Virtual_Controllers/L4_MABX/L4_Controller/Task_10ms/STEERCTRL_10ms/PID/PID ==
  Err : Inport
  Kp : Inport  Port=2
  Ti : Inport  Port=3
  Td : Inport  Port=4
  Reset_f : Inport  Port=5
  Ts : Inport  Port=6
  UpperLim : Inport  Port=7
  LowerLim : Inport  Port=8
  InitOutput : Inport  Port=9
  Constant : Constant  Value=0
  Constant2 : Constant  Value=-1
  Constant3 : Constant
  PID : Subsystem
  Relational Operator : RelationalOperator  OutDataTypeStr=boolean  RndMeth=Nearest
  Relational Operator1 : RelationalOperator  Operator=<=  OutDataTypeStr=boolean  RndMeth=Nearest
  Saturation Dynamic : simulink/Discontinuities/Saturation Dynamic  RequirementInfo={} %GIDa_a8a084d7_bda8_4443_856d_eb85f2a73d9b  OutMin=[]  OutMax=[]  OutDataTypeStr=Inherit: Same as second input  OutDataType=sfix(16)  OutScaling=2^-10  DoSatur=off
  Switch : Switch  Criteria=u2 ~= 0
  Switch1 : Switch  Criteria=u2 ~= 0
  Unit Delay : UnitDelay  SampleTime=-1
  Y : Outport
  P : Outport  Port=2
  I : Outport  Port=3
  D : Outport  Port=4
  wires:
  Saturation Dynamic/1 -> Y/1
  PID/1(Out1) -> Unit Delay/1, Saturation Dynamic/2
  Err/1 -> PID/3(Err)
  Ts/1 -> PID/7(Ts)
  Td/1 -> PID/6(Td)
  Ti/1 -> PID/5(Ti)
  Kp/1 -> PID/4(K)
  InitOutput/1 -> PID/1(Init)
  PID/2(P_Out) -> P/1
  PID/3(I_Out) -> I/1
  PID/4(D_Out1) -> D/1
  Relational Operator1/1 -> Switch1/2
  Constant/1 -> Switch1/3
  Constant2/1 -> Switch1/1
  Switch1/1 -> Switch/3
  Constant3/1 -> Switch/1
  Switch/1 -> PID/8(Sat_state)
  Relational Operator/1 -> Switch/2
  UpperLim/1 -> Saturation Dynamic/1, Relational Operator/2
  LowerLim/1 -> Saturation Dynamic/3, Relational Operator1/2
  Unit Delay/1 -> Relational Operator/1, Relational Operator1/1
  Reset_f/1 -> PID/2(Reset_Integral)

== system L4_SIM/Controllers/Virtual_Controllers/L4_MABX/L4_Controller/Task_10ms/Vehicle_speed_target/Determine_linear_vehicle_speed_profile/Determine_slew_time_values ==
  F_Reset : Inport
  Vehicle_speed : Inport  Port=2
  Vehicle_speed_target : Inport  Port=3
  Distance_m : Inport  Port=4
  dT : Inport  Port=5
  Abs2 : EmE_MBD_Blockset/Math Operators/Abs
      settings: SourceProductName=PACCAR EmE MBD Blockset
  Bus Creator : BusCreator  Inputs=3
  Bus Selector1 : BusSelector  OutputSignals=Vehicle_speed_target,Vehicle_speed,Distance_m
  Divide : Product  Inputs=*/  InputSameDT=on
  Divide2 : Product  Inputs=*/  InputSameDT=on
  Gain2 : Gain  Gain=1/3.6
  If_Then_Else : EmE_MBD_Blockset/Signal Routing/If_Then_Else
      settings: SourceProductName=PACCAR EmE MBD Blockset
  MinMax3 : MinMax  Function=max  Inputs=2  InputSameDT=on
  Saturation1 : Saturate  UpperLimit=Inf  LowerLimit=0.001
      settings: AttributesFormatString=|
      | Min: %<LowerLimit>
      | Max: %<UpperLimit>
  Saturation4 : Saturate  UpperLimit=255  LowerLimit=0.001
      settings: AttributesFormatString=|
      | Min: %<LowerLimit>
      | Max: %<UpperLimit>
  Subtract : Sum  Inputs=-+  InputSameDT=on
  Unit_Delay : UnitDelay  SampleTime=-1
      settings: AttributesFormatString=IC: %<vinit>
  Inc : Outport
  Dec : Outport  Port=2
  wires:
  Bus Selector1/2 -> Gain2/1, Subtract/2  "<Vehicle_speed>"
  Bus Selector1/3 -> Divide2/1  "<Distance_m>"
  Subtract/1 -> Abs2/1  "err"
  Gain2/1 -> Saturation4/1
  Divide2/1 -> MinMax3/1  "time_to_target_vspd_secs"
  Bus Selector1/1 -> Subtract/1  "<Vehicle_speed_target>"
  dT/1 -> MinMax3/2
  Saturation4/1 -> Divide2/2
  MinMax3/1 -> Saturation1/1
  Abs2/1 -> Divide/1  "err_abs"
  Divide/1 -> Dec/1, Inc/1
  Saturation1/1 -> Divide/2
  Bus Creator/1 -> If_Then_Else/2
  If_Then_Else/1 -> Unit_Delay/1, Bus Selector1/1
  Unit_Delay/1 -> If_Then_Else/3
  Distance_m/1 -> Bus Creator/3  "Distance_m"
  Vehicle_speed_target/1 -> Bus Creator/1  "Vehicle_speed_target"
  Vehicle_speed/1 -> Bus Creator/2  "Vehicle_speed"
  F_Reset/1 -> If_Then_Else/1

== system L4_SIM/Controllers/Virtual_Controllers/L4_MABX/L4_Controller/Task_10ms/Vehicle_speed_target/Determine_sigmoid_vehicle_speed_profile/Determine_inhibit_sigmoid_vehicle_speed_profile ==
  F_Enable : Inport
  Distance_m : Inport  Port=2
  Vehicle_speed : Inport  Port=3
  Vehicle_speed_target : Inport  Port=4
  Position_vector_m : Inport  Port=5
  Vehicle_speed_vector_kph : Inport  Port=6
  Acceleration_vector_ms2 : Inport  Port=7
  Jerk_vector_ms3 : Inport  Port=8
  ACCEL_RATE_ABS_MAX_THRESHOLD_MS2_APV : EmE_MBD_Blockset/Sources/APV  conval=5
      settings: SourceProductName=PACCAR EmE MBD Blockset
  ACCEL_RATE_ABS_MIN_THRESHOLD_MS2_APV : EmE_MBD_Blockset/Sources/APV  conval=-5
      settings: SourceProductName=PACCAR EmE MBD Blockset
  Abs : EmE_MBD_Blockset/Math Operators/Abs
      settings: SourceProductName=PACCAR EmE MBD Blockset
  Abs1 : EmE_MBD_Blockset/Math Operators/Abs
      settings: SourceProductName=PACCAR EmE MBD Blockset
  Abs2 : EmE_MBD_Blockset/Math Operators/Abs
      settings: SourceProductName=PACCAR EmE MBD Blockset
  CPV : EmE_MBD_Blockset/Sources/CPV  conval=false
      settings: SourceProductName=PACCAR EmE MBD Blockset
  Capture_initial_vehicle_speed_value : Subsystem
  Compare To Zero : simulink/Logic and Bit Operations/Compare To Zero  relop=<  OutDataTypeStr=boolean
  JERK_RATE_ABS_MAX_THRESHOLD_MS3_APV : EmE_MBD_Blockset/Sources/APV  conval=5
      settings: SourceProductName=PACCAR EmE MBD Blockset
  JERK_RATE_ABS_MIN_THRESHOLD_MS3_APV : EmE_MBD_Blockset/Sources/APV  conval=-5
      settings: SourceProductName=PACCAR EmE MBD Blockset
  Logical Operator : EmE_MBD_Blockset/Logic and Bit Operations/Logical Operator  Operator=OR  Inputs=1
      settings: SourceProductName=PACCAR EmE MBD Blockset
  Logical Operator1 : EmE_MBD_Blockset/Logic and Bit Operations/Logical Operator  Operator=AND  Inputs=2
      settings: SourceProductName=PACCAR EmE MBD Blockset
  Logical Operator2 : EmE_MBD_Blockset/Logic and Bit Operations/Logical Operator  Operator=AND  Inputs=2
      settings: SourceProductName=PACCAR EmE MBD Blockset
  Logical Operator3 : EmE_MBD_Blockset/Logic and Bit Operations/Logical Operator  Operator=AND  Inputs=2
      settings: SourceProductName=PACCAR EmE MBD Blockset
  Logical Operator4 : Logic  Operator=OR  Inputs=8  AllPortsSameDT=off  OutDataTypeStr=boolean
  MAX_DISTANCE_DELTA_THRESHOLD_M_APV : EmE_MBD_Blockset/Sources/APV  conval=0.5
      settings: SourceProductName=PACCAR EmE MBD Blockset
  MAX_VSPD_DELTA_THRESHOLD_KPH_APV : EmE_MBD_Blockset/Sources/APV  conval=5
      settings: SourceProductName=PACCAR EmE MBD Blockset
  MIN_VSPD_DELTA_THRESHOLD_KPH_APV : EmE_MBD_Blockset/Sources/APV  conval=5
      settings: SourceProductName=PACCAR EmE MBD Blockset
  MinMax10 : MinMax  Function=max  InputSameDT=on
  MinMax3 : MinMax  InputSameDT=on
  MinMax4 : MinMax  Function=max  InputSameDT=on
  MinMax5 : MinMax  Inputs=2  InputSameDT=on
  MinMax6 : MinMax  Function=max  Inputs=2  InputSameDT=on
  MinMax7 : MinMax  InputSameDT=on
  MinMax8 : MinMax  Function=max  InputSameDT=on
  MinMax9 : MinMax  InputSameDT=on
  Relational Operator{,1..2,4,6} (5 alike) : EmE_MBD_Blockset/Logic and Bit Operations/Relational Operator  func=>
      settings: SourceProductName=PACCAR EmE MBD Blockset
  Relational Operator3 : EmE_MBD_Blockset/Logic and Bit Operations/Relational Operator  func=<
      settings: SourceProductName=PACCAR EmE MBD Blockset
  Relational Operator5 : EmE_MBD_Blockset/Logic and Bit Operations/Relational Operator  func=<
      settings: SourceProductName=PACCAR EmE MBD Blockset
  SR flip-flop : EmE_MBD_Blockset/Logic and Bit Operations/SR flip-flop
      settings: SourceProductName=PACCAR EmE MBD Blockset
  Selector : Selector  InputPortWidth=33  IndexOptions=Index vector (dialog)  Indices=33  OutputSizes=1
  Subtract : Sum  Inputs=+-  InputSameDT=on
  Subtract1 : Sum  Inputs=+-  InputSameDT=on
  Subtract2 : Sum  Inputs=+-  InputSameDT=on
  Terminator : Terminator
  F_Inhibit_sigmoid_vector_shaping : Outport  LibraryBlock=EmE_MBD_Blockset/Sinks/Out  OutputWhenDisabled=reset
  Vehicle_speed_initial : Outport  Port=2
  wires:
  Relational Operator6/1 -> Logical Operator3/1
  Position_vector_m/1 -> Selector/1
  Selector/1 -> Subtract2/2
  Logical Operator3/1 -> Logical Operator4/8  "f_distance_max_delta_greater_than_threshold"
  Distance_m/1 -> Subtract2/1
  Subtract2/1 -> Abs2/1
  Abs2/1 -> Relational Operator6/1
  MAX_DISTANCE_DELTA_THRESHOLD_M_APV/1 -> Relational Operator6/2
  Vehicle_speed/1 -> Capture_initial_vehicle_speed_value/1(Vehicle_speed)
  Capture_initial_vehicle_speed_value/1(Vehicle_speed_initial) -> MinMax5/1, MinMax6/1, Vehicle_speed_initial/1
  Vehicle_speed_target/1 -> MinMax6/2, MinMax5/2
  MinMax6/1 -> Subtract1/2
  MinMax5/1 -> Subtract/2
  Subtract/1 -> Abs/1
  Subtract1/1 -> Abs1/1
  Relational Operator1/1 -> Logical Operator1/1
  MAX_VSPD_DELTA_THRESHOLD_KPH_APV/1 -> Relational Operator1/2
  Logical Operator2/1 -> Logical Operator4/2  "f_vspd_min_delta_greater_than_threshold"
  MinMax9/1 -> Relational Operator5/1
  JERK_RATE_ABS_MIN_THRESHOLD_MS3_APV/1 -> Relational Operator5/2
  Logical Operator/1 -> Logical Operator4/1  "f_vspd_output_less_than_zero"
  MinMax4/1 -> Subtract1/1
  MIN_VSPD_DELTA_THRESHOLD_KPH_APV/1 -> Relational Operator/2
  Jerk_vector_ms3/1 -> MinMax10/1, MinMax9/1
  Abs1/1 -> Relational Operator1/1
  Abs/1 -> Relational Operator/1
  Logical Operator1/1 -> Logical Operator4/3  "f_vspd_max_delta_greater_than_threshold"
  Relational Operator5/1 -> Logical Operator4/7  "f_jerk_rate_greater_than_threshold"
  MinMax10/1 -> Relational Operator4/1
  ACCEL_RATE_ABS_MAX_THRESHOLD_MS2_APV/1 -> Relational Operator2/2
  MinMax8/1 -> Relational Operator2/1
  Relational Operator/1 -> Logical Operator2/1
  JERK_RATE_ABS_MAX_THRESHOLD_MS3_APV/1 -> Relational Operator4/2
  Acceleration_vector_ms2/1 -> MinMax8/1, MinMax7/1
  Vehicle_speed_vector_kph/1 -> Compare To Zero/1, MinMax3/1, MinMax4/1
  Relational Operator2/1 -> Logical Operator4/4  "f_accel_rate_greater_than_threshold"
  Relational Operator3/1 -> Logical Operator4/5  "f_decel_rate_greater_than_threshold"
  MinMax3/1 -> Subtract/1
  SR flip-flop/1 -> Logical Operator2/2, Logical Operator1/2, Logical Operator3/2
  MinMax7/1 -> Relational Operator3/1
  SR flip-flop/2 -> Terminator/1
  Relational Operator4/1 -> Logical Operator4/6  "f_jerk_rate_greater_than_threshold"
  CPV/1 -> SR flip-flop/2
  Logical Operator4/1 -> F_Inhibit_sigmoid_vector_shaping/1  "F_Inhibit_sigmoid_vector_shaping"
  ACCEL_RATE_ABS_MIN_THRESHOLD_MS2_APV/1 -> Relational Operator3/2
  F_Enable/1 -> Capture_initial_vehicle_speed_value/2(F_Enable), SR flip-flop/1
  Compare To Zero/1 -> Logical Operator/1
